simulink model "PILAN2021a"  (R2021a)
settings: Solver=FixedStepAuto  StartTime=0.0  StopTime=41.24  FixedStep=0.001  RelTol=1e-3  EnableMultiTasking=on
values from neighbouring files (symbols this model uses):
  den_lpf_d = den_lpf20    [Mainframe_init.m]    (also in load_autopilot.m)
  Emulated_FCC_IO_Delay = 7    [Mainframe_init.m]
  Enable_Gyros = 0    [Mainframe_init.m]
  Enable_INS = 0    [Mainframe_init.m]
  num_lpf_d = num_lpf20    [Mainframe_init.m]    (also in load_autopilot.m)
undefined symbols (not defined in the file or in its folder): act_dmp, act_omega, Actuator, Aerodynamics, aMode, Autopilot, AUX, c_b_WGS, c_be, c_flat, c_grav, c_h_geop0, c_h_geope, c_pa0, c_pe, c_r0, c_rot, c_rsma, c_Tmp0, d_siB_0, d_siB_max, d_siB_min, dd_siB_max, dd_siB_min, dev, DiscIntNeverNeededParam, e_pa, e_Tmp, Earth, fin_maxrate, flag_I_act_switch, flag_I_aero_switch, flag_I_flat, flag_I_gravity_switch, flag_I_rot, Flight_Logic, hcr, HIL_Data, JMMM_0, JMMM_e, JSPB_e, lat_0, lon_0, Mass_Props, mB_0, mM_0, mM_e, National_Instruments, pBII_0, PCIe, pMPB, pNPB, propellant_kg, prp_FBPB, prp_mdot, prp_T, pSPB, pwm_output1, qEG_0, qIB_0 ... (+30)
libraries: simulink x42, simulink_extras x24, aerolibcommonsys x4, px4lib x2, custom_blocks x1, dspstat3 x1, pil_lib x1, aerolibtransform2 x1, sldrtlib x1, aerolibnav x1
(part 1 of 16)
settings Model: CodeVerificationMode=processor-in-the-loop (pil)  ExtModeTrigDuration=10  Creator=m.hiepp  LastModifiedBy=sasson
settings SolverCC: AlgebraicLoopSolver=TrustRegion  PositivePriorityOrder=on  AutoInsertRateTranBlk=on
settings DataIOCC: SignalLogging=off  ReturnWorkspaceOutputs=off
settings OptimizationCC: EnhancedBackFolding=on  PassReuseOutputArgsAs=Individual arguments  ZeroExternalMemoryAtStartup=off  ZeroInternalMemoryAtStartup=off  MaxStackSize=64  OptimizeBlockOrder=speed  DifferentSizesBufferReuse=on  OptimizationCustomize=off  EfficientTunableParamExpr=on
settings DebuggingCC: ParameterPrecisionLossMsg=none  ParameterTunabilityLossMsg=error  SFMachineParentedDataDiag=warning  UnderSpecifiedDimensionMsg=warning  ArithmeticOperatorsInVariantConditions=warning
settings HardwareCC: ProdBitPerPointer=32  ProdBitPerSizeT=32  ProdBitPerPtrDiffT=32  ProdLargestAtomicInteger=Long  ProdLargestAtomicFloat=Double  ProdWordSize=32  ProdLongLongMode=on  ProdHWDeviceType=ARM Compatible->ARM Cortex
settings SFSimCC: MATLABDynamicMemAlloc=off  CustomCodeUndefinedFunction=UseInterfaceOnly  SimTargetLang=C++
settings RTWCC: SystemTargetFile=ert.tlc  HardwareBoard=PX4 Pixhawk 2.1 (Cube)  TLCOptions="-aInlineSetEventsForThisBaseRateFcn=TLC_FALSE -aSuppressMultiTaskScheduler=TLC_FALSE  -aRateBasedStepFcn=0"  TemplateMakefile=ert_default_tmf  GenerateReport=on  Toolchain=GNU Tools for PX4 Autopilots  IncludeHyperlinkInReport=on  LaunchReport=on  PortableWordSizes=on  CreateSILPILBlock=PIL  TargetLang=C++  GenerateTraceInfo=on  GenerateTraceReport=on  GenerateTraceReportSl=on  GenerateTraceReportSf=on  GenerateTraceReportEml=on
settings CodeAppCC: ForceParamTrailComments=on  IgnoreCustomStorageClasses=off  MaxIdLength=95  OperatorAnnotations=on  SimulinkDataObjDesc=on  SFDataObjDesc=on  InsertBlockDesc=on
settings ERTTargetCC: SupportContinuousTime=on  ExtModeTransport=3  ExtModeStaticAlloc=on  ExtModeStaticAllocSize=1024  ExtModeMexFile=ext_xcp  ExtModeIntrfLevel=Level2 - Open

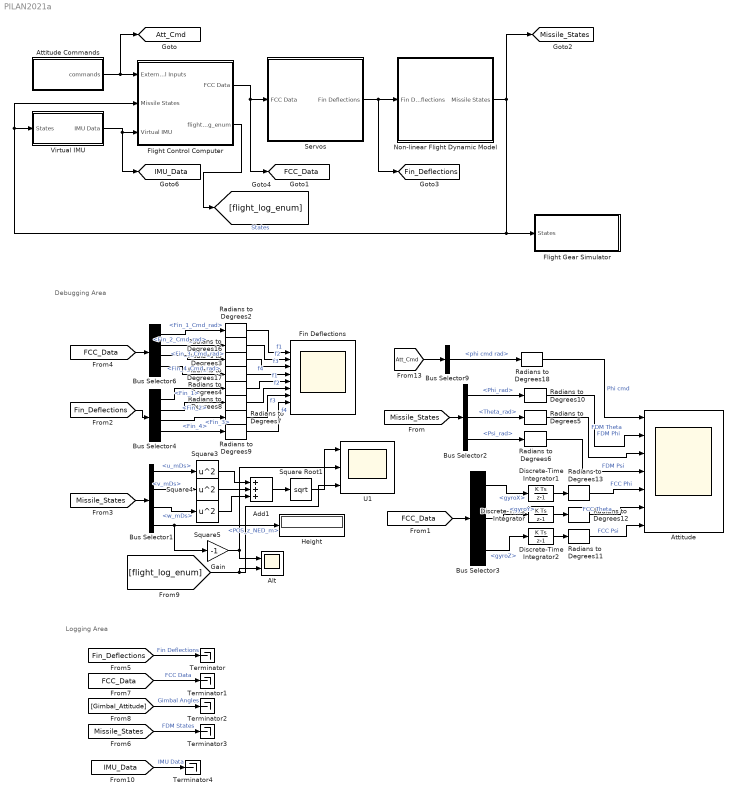
== system PILAN2021a ==
  note: Debugging Area
  note: Logging Area
  Add1 : Sum  Inputs=+++
  Alt : Scope  NumInputPorts=2
  Attitude : Scope  NumInputPorts=7
  Attitude Commands : Subsystem
  Bus Selector1 : BusSelector  OutputSignals=Translation_States.u_mDs,Translation_States.v_mDs,Translation_States.w_mDs,POS_NED.POS_z_NED_m
  Bus Selector2 : BusSelector  OutputSignals=Attitude_States.ATT_Euler.Phi_rad,Attitude_States.ATT_Euler.Theta_rad,Attitude_States.ATT_Euler.Psi_rad
  Bus Selector3 : BusSelector  OutputSignals=Internal Data.gyroX,Internal Data.gyroY,Internal Data.gyroZ
  Bus Selector4 : BusSelector  OutputSignals=Fin_1,Fin_2,Fin_3,Fin_4
  Bus Selector6 : BusSelector  OutputSignals=Control Surface Cmd.Fin_1_Cmd_rad,Control Surface Cmd.Fin_2_Cmd_rad,Control Surface Cmd.Fin_3_Cmd_rad,Control Surface Cmd.Fin_4_Cmd_rad
  Bus Selector9 : BusSelector  OutputSignals=phi cmd rad
  Discrete-Time Integrator : DiscreteIntegrator  SampleTime=0.01  ICPrevOutput=DiscIntNeverNeededParam  ICPrevScaledInput=DiscIntNeverNeededParam
  Discrete-Time Integrator1 : DiscreteIntegrator  SampleTime=0.01  ICPrevOutput=DiscIntNeverNeededParam  ICPrevScaledInput=DiscIntNeverNeededParam
  Discrete-Time Integrator2 : DiscreteIntegrator  SampleTime=0.01  ICPrevOutput=DiscIntNeverNeededParam  ICPrevScaledInput=DiscIntNeverNeededParam
  Fin Deflections : Scope  NumInputPorts=8
  Flight Control Computer : Subsystem  VariantControl=VSS_FCC_REAL
  Flight Gear Simulator : Subsystem  Variant=on
  Gain : Gain  Gain=-1
  Height : Display
  Non-linear Flight Dynamic Model : Subsystem  VariantControl=VSS_FDM_SOPH
      mask init:
      | load('generated_FDM_params')
  Radians to Degrees{2..13,16..18} (15 alike) : simulink_extras/Transformations/Radians to Degrees
  Servos : Subsystem  Variant=on
  Square Root1 : Sqrt  SaturateOnIntegerOverflow=on
  Square3 : Math  Operator=square  SaturateOnIntegerOverflow=on
  Square4 : Math  Operator=square  SaturateOnIntegerOverflow=on
  Square5 : Math  Operator=square  SaturateOnIntegerOverflow=on
  Terminator{,1..4} (5 alike) : Terminator
  U1 : Scope  NumInputPorts=3
  Virtual IMU : Subsystem
  tag scope: Att_Cmd=global, FCC_Data=global, Fin_Deflections=global, IMU_Data=global, Missile_States=global
  wires:
  [IMU_Data] -> Terminator4/1  "IMU Data"
  Bus Selector3/2 -> Discrete-Time Integrator/1  "<gyroY>"
  Discrete-Time Integrator1/1 -> Radians to Degrees13/1
  Radians to Degrees11/1 -> Attitude/7  "FCC Psi"
  Discrete-Time Integrator/1 -> Radians to Degrees12/1
  [FCC_Data] -> Bus Selector6/1
  Bus Selector1/4 -> Gain/1, Height/1  "<POS_z_NED_m>"
  Flight Control Computer/1(FCC Data) -> [FCC_Data], Servos/1(FCC Data)
  Radians to Degrees2/1 -> Fin Deflections/1  "f1"
  Radians to Degrees4/1 -> Fin Deflections/5  "f1"
  Radians to Degrees18/1 -> Attitude/1  "Phi cmd"
  Bus Selector6/1 -> Radians to Degrees2/1  "<Fin_1_Cmd_rad>"
  Radians to Degrees3/1 -> Fin Deflections/3  "f3"
  Radians to Degrees17/1 -> Fin Deflections/4  "f4"
  Radians to Degrees13/1 -> Attitude/5  "FCC Phi"
  [Missile_States] -> Bus Selector1/1
  Bus Selector3/1 -> Discrete-Time Integrator1/1  "<gyroX>"
  Discrete-Time Integrator2/1 -> Radians to Degrees11/1
  [Gimbal_Attitude] -> Terminator2/1  "Gimbal Angles"
  [FCC_Data] -> Terminator1/1  "FCC Data"
  Square5/1 -> Add1/3
  Bus Selector6/2 -> Radians to Degrees16/1  "<Fin_2_Cmd_rad>"
  [Fin_Deflections] -> Terminator/1  "Fin Deflections"
  Bus Selector6/4 -> Radians to Degrees17/1  "<Fin_4_Cmd_rad>"
  Square3/1 -> Add1/1
  Bus Selector1/1 -> Square3/1  "<u_mDs>"
  Add1/1 -> Square Root1/1
  Radians to Degrees6/1 -> Attitude/4  "FDM Psi"
  Bus Selector4/4 -> Radians to Degrees9/1  "<Fin_4>"
  Virtual IMU/1(" IMU Data") -> [IMU_Data], Flight Control Computer/3(Virtual IMU)
  Radians to Degrees10/1 -> Attitude/2  "FDM Phi"
  Bus Selector1/3 -> Square5/1  "<w_mDs>"
  Bus Selector1/2 -> Square4/1  "<v_mDs>"
  Radians to Degrees5/1 -> Attitude/3  "FDM Theta"
  Non-linear Flight Dynamic Model/1(Missile States) -> Flight Control Computer/2(Missile States), Virtual IMU/1(States), Flight Gear Simulator/1(States), [Missile_States]  "States"
  Bus Selector9/1 -> Radians to Degrees18/1  "<phi cmd rad>"
  Square4/1 -> Add1/2
  [Missile_States] -> Bus Selector2/1
  Bus Selector2/2 -> Radians to Degrees5/1  "<Theta_rad>"
  Bus Selector6/3 -> Radians to Degrees3/1  "<Fin_3_Cmd_rad>"
  Servos/1(Fin Deflections) -> [Fin_Deflections], Non-linear Flight Dynamic Model/1(Fin Deflections)
  Radians to Degrees16/1 -> Fin Deflections/2  "f2"
  Radians to Degrees9/1 -> Fin Deflections/8  "f4"
  Attitude Commands/1(commands) -> [Att_Cmd], Flight Control Computer/1(External Inputs)
  Radians to Degrees8/1 -> Fin Deflections/6  "f2"
  Bus Selector3/3 -> Discrete-Time Integrator2/1  "<gyroZ>"
  Bus Selector2/3 -> Radians to Degrees6/1  "<Psi_rad>"
  Bus Selector4/3 -> Radians to Degrees7/1  "<Fin_3>"
  Radians to Degrees7/1 -> Fin Deflections/7  "f3"
  Bus Selector2/1 -> Radians to Degrees10/1  "<Phi_rad>"
  [Att_Cmd] -> Bus Selector9/1
  [Missile_States] -> Terminator3/1  "FDM States"
  [Fin_Deflections] -> Bus Selector4/1
  Radians to Degrees12/1 -> Attitude/6  "FCC Theta"
  Bus Selector4/1 -> Radians to Degrees4/1  "<Fin_1>"
  [FCC_Data] -> Bus Selector3/1
  Square Root1/1 -> U1/1
  Bus Selector4/2 -> Radians to Degrees8/1  "<Fin_2>"
  Gain/1 -> Alt/1, U1/2
  Flight Control Computer/2(flight_log_enum) -> [flight_log_enum]
  [flight_log_enum] -> U1/3, Alt/2

== system PILAN2021a/Attitude Commands ==
  Bus Creator : BusCreator  Inputs=3
  Delayed Sine : custom_blocks/Delayed Sine  amp=deg2rad(65)  bias=0  freq=pi/3  phase=0  onTime=5  duration=3
  Enabled Subsystem1 : Subsystem  TreatAsAtomicUnit=on
  Radians to Degrees : simulink_extras/Transformations/Radians to Degrees
  Scope : Scope
  Zero : Constant  Value=0  OutDataTypeStr=Inherit: Inherit via back propagation
  Zero1 : Constant  Value=0  OutDataTypeStr=Inherit: Inherit via back propagation
  commands : Outport
  wires:
  Delayed Sine/1 -> Radians to Degrees/1, Bus Creator/1  "phi cmd rad"
  Bus Creator/1 -> commands/1
  Zero/1 -> Bus Creator/3  "psi cmd rad"
  Zero1/1 -> Bus Creator/2  "theta cmd rad"
  Enabled Subsystem1/1(CalibrationTime) -> Delayed Sine/1  "Calibration Time"
  [HIL_Ready] -> Enabled Subsystem1/Trigger
  Radians to Degrees/1 -> Scope/1

== system PILAN2021a/Flight Control Computer ==
  External Inputs : Inport
  Missile States : Inport  Port=2
  Virtual IMU : Inport  Port=3
  Bus Creator : BusCreator  Inputs=2
  Bus Selector : BusSelector  OutputSignals=signal1,flight_mode_enum
  Constant1 : Constant  Value=Enable_Gyros  OutDataTypeStr=single
  Constant4 : Constant  Value=Enable_INS  OutDataTypeStr=single
  Debug : Scope
  FCC - Real or Emulated : Subsystem  Variant=on
  FCC_SYNC : Scope
  Heartbeat Check : Subsystem
  Recieve from FCC : Subsystem
  Send to FCC : Subsystem
  FCC Data : Outport
  flight_log_enum : Outport  Port=2
  wires:
  Constant4/1 -> Send to FCC/1(Enable INS Flag)
  Recieve from FCC/2(internal data) -> Bus Creator/2  "Internal Data"
  Recieve from FCC/1(fin_cmd_rad) -> Bus Creator/1  "Control Surface Cmd"
  External Inputs/1 -> Send to FCC/5(External Inputs)
  Missile States/1 -> Send to FCC/3(Missile States)
  Send to FCC/1(data out) -> FCC - Real or Emulated/1(Input Data)
  Recieve from FCC/3(Other) -> Debug/1
  Constant1/1 -> Send to FCC/2(Enable Gyros Flag)
  Heartbeat Check/1(Communication Delay) -> FCC_SYNC/1
  Bus Creator/1 -> FCC Data/1  "FCC data"
  Virtual IMU/1 -> Send to FCC/4(Virtual IMU)
  Send to FCC/2(Heartbeat Send) -> [Heartbeat_Sent]
  Recieve from FCC/4(HeartBeat_recived) -> [Heartbeat_Received]
  [Heartbeat_Sent] -> Heartbeat Check/1(Send)
  [Heartbeat_Received] -> Heartbeat Check/2(receive)  "receive"
  FCC - Real or Emulated/1(Output Data) -> Bus Selector/1
  Bus Selector/1 -> Recieve from FCC/1(data in)  "<signal1>"
  Bus Selector/2 -> flight_log_enum/1  "<flight_mode_enum>"

== system PILAN2021a/Flight Gear Simulator ==
  States : Inport
  Flight Simulator Off : Subsystem  VariantControl=VSS_FLIGHTGEAR_OFF
  Flight Simulator On : Subsystem  VariantControl=VSS_FLIGHTGEAR_ON

== system PILAN2021a/Non-linear Flight Dynamic Model ==
  Fin Deflections : Inport
  Environment : Subsystem
  Extract States : Subsystem
  GRM_Airframe : Subsystem
      mask Display: image('$imagefile'); % Use "Edit Image" on toolstrip to change.
  Stop-Condition : Subsystem
  Subsystem1 : Subsystem  Commented=on
  Translate Fins : Subsystem
  Missile States : Outport  VectorParamsAs1DForOutWhenUnconnected=off
  wires:
  Fin Deflections/1 -> Translate Fins/1(Servo Deflections)
  Extract States/1(States) -> Missile States/1, Stop-Condition/1(States)  "States"
  Translate Fins/1(afinB) -> GRM_Airframe/1(siB_cmd)
  GRM_Airframe/1(airfr) -> Extract States/1(airfr_bus)
  Environment/1(env_glbl_bus) -> GRM_Airframe/2(T_sim_glbl)

== system PILAN2021a/Servos ==
  FCC Data : Inport
  Emulated Servos : Subsystem  VariantControl=VSS_SERVOS_OFF
  Real Servos : Subsystem  VariantControl=VSS_SERVOS_ON
  Fin Deflections : Outport

== system PILAN2021a/Virtual IMU ==
  States : Inport
  Bus Creator1 : BusCreator  Inputs=3
  Bus Creator10 : BusCreator  Inputs=2
  Bus Creator2 : BusCreator  Inputs=3
  Bus Selector : BusSelector  OutputSignals=Translation_States_Dot.u_dot_mDs2,Translation_States_Dot.v_dot_mDs2,Translation_States_Dot.w_dot_mDs2,Rotation_States.p_radDs,Rotation_States.q_radDs,Rotation_States.r_radDs,Rotation_States_Dot.p_dot_radDs2,Rotation_States_Dot.q_dot_radDs2,Rotation_States_Dot.r_dot_radDs2,Attitude_States.ATT_Euler.Phi_rad,Attitude_States.ATT_Euler.Theta_rad
  Constant1 : Constant  Value=[0,0,0]
  Demux8 : Demux  Outputs=3
  Demux9 : Demux  Outputs=3
  Gravity Vector : Subsystem
  Mux1 : Mux  Inputs=3
  Mux2 : Mux  Inputs=3
  Mux3 : Mux  Inputs=3
  Three-axis Inertial Measurement Unit : aerolibnav/Three-axis Inertial Measurement Unit  units=Metric (MKS)  imu=[0.43197 -0.00245 -0.01265]  i_Ts=0  dtype_a=on  w_a=190  z_a=0.707  a_sf_cc=[1.00135 0.0029375 0.00018125; -0.0029375 1.001525 0.0025625; -0.00018125 -0.0025625 1.004375]  a_bias=[0.086853 0.0258 -0.009194]  a_sat="[-156.921  -156.921  -156.921  156.921 156.921 156.921]"  dtype_g=on  w_g=190  z_g=0.707  g_sf_cc=[1.0045125 0.0045875 -0.005975; -0.0045875 1.0017125 0.0036875; 0.005975 -0.0036875 1.00243125]  g_bias=[-0.02167 0.011301 0.00202676]  g_sens=[0.000062068 0.0000443968 -0.0010608]  g_sat="[-34.9  -34.9  -34.9  34.9 34.9 34.9]"  i_rand=off  i_seeds=[23093 23094 23095 23096 23097 23098]  i_pow=[0.001 0.001 0.001 0.0001 0.0001 0.0001]
  " IMU Data" : Outport  VectorParamsAs1DForOutWhenUnconnected=off
  wires:
  Bus Selector/5 -> Mux2/2  "<q_radDs>"
  Mux3/1 -> Three-axis Inertial Measurement Unit/3
  Bus Selector/3 -> Mux1/3  "<w_dot_mDs2>"
  Bus Creator10/1 -> " IMU Data"/1  "Virtual IMU"
  Bus Selector/6 -> Mux2/3  "<r_radDs>"
  States/1 -> Bus Selector/1
  Bus Selector/11 -> Gravity Vector/2(Theta)  "<Theta_rad>"
  Bus Selector/2 -> Mux1/2  "<v_dot_mDs2>"
  Three-axis Inertial Measurement Unit/2 -> Demux9/1
  Bus Creator2/1 -> Bus Creator10/2  "gyro"
  Mux1/1 -> Three-axis Inertial Measurement Unit/1
  Mux2/1 -> Three-axis Inertial Measurement Unit/2
  Demux8/3 -> Bus Creator1/3  "accZ"
  Demux9/2 -> Bus Creator2/2  "gyroY"
  Demux9/1 -> Bus Creator2/1  "gyroX"
  Three-axis Inertial Measurement Unit/1 -> Demux8/1
  Demux8/1 -> Bus Creator1/1  "accX"
  Constant1/1 -> Three-axis Inertial Measurement Unit/4
  Bus Selector/4 -> Mux2/1  "<p_radDs>"
  Bus Creator1/1 -> Bus Creator10/1  "accelerometer"
  Demux8/2 -> Bus Creator1/2  "accY"
  Bus Selector/1 -> Mux1/1  "<u_dot_mDs2>"
  Gravity Vector/1(g) -> Three-axis Inertial Measurement Unit/5
  Demux9/3 -> Bus Creator2/3  "gyroZ"
  Bus Selector/10 -> Gravity Vector/1(Phi)  "<Phi_rad>"
  Bus Selector/8 -> Mux3/2  "<q_dot_radDs2>"
  Bus Selector/7 -> Mux3/1  "<p_dot_radDs2>"
  Bus Selector/9 -> Mux3/3  "<r_dot_radDs2>"

== system PILAN2021a/Attitude Commands/Enabled Subsystem1 ==
  Trigger : TriggerPort  VariantControl=Variant  PortDimensions=1
  Digital Clock : DigitalClock  SampleTime=-1
  CalibrationTime : Outport  InitialOutput=1e9
  wires:
  Digital Clock/1 -> CalibrationTime/1

== system PILAN2021a/Flight Control Computer/FCC - Real or Emulated ==
  Input Data : Inport
  Emulated FCC : Subsystem  VariantControl=VSS_FCC_EMUL
  Real FCC : Subsystem  VariantControl=VSS_FCC_REAL
  Output Data : Outport

== system PILAN2021a/Flight Control Computer/Heartbeat Check ==
  note: This block ensures the Pixhawk is connected and functioning correctly
  Send : Inport
  receive : Inport  Port=2
  In Sync : Subsystem
  Communication Delay : Outport
  wires:
  Send/1 -> In Sync/1(send)
  receive/1 -> In Sync/2(receive)
  In Sync/1(Heartbeat Sync) -> Communication Delay/1

== system PILAN2021a/Flight Control Computer/Recieve from FCC ==
  data in : Inport
  Bus Creator1 : BusCreator  Inputs=12
  Bus Creator4 : BusCreator  Inputs=4
  Cast To Double{,1..17} (18 alike) : DataTypeConversion  OutDataTypeStr=double
  Demux : Demux  Outputs=18
  fin_cmd_rad : Outport  PortDimensions=4
  internal data : Outport  Port=2
  Other : Outport  Port=3
  HeartBeat_recived : Outport  Port=4
  wires:
  data in/1 -> Demux/1
  Demux/1 -> Cast To Double/1
  Demux/7 -> Cast To Double6/1  "gyroY"
  Demux/11 -> Cast To Double10/1  "w"
  Demux/10 -> Cast To Double9/1  "v"
  Demux/9 -> Cast To Double8/1  "u"
  Demux/8 -> Cast To Double7/1  "gyroZ"
  Demux/4 -> Cast To Double3/1  "Fin_3_Cmd_rad"
  Demux/5 -> Cast To Double4/1  "Fin_4_Cmd_rad"
  Demux/3 -> Cast To Double2/1  "Fin_2_Cmd_rad"
  Demux/2 -> Cast To Double1/1  "Fin_1_Cmd_rad"
  Demux/6 -> Cast To Double5/1  "gyroX"
  Bus Creator4/1 -> fin_cmd_rad/1
  Bus Creator1/1 -> internal data/1
  Cast To Double1/1 -> Bus Creator4/1  "Fin_1_Cmd_rad"
  Cast To Double2/1 -> Bus Creator4/2  "Fin_2_Cmd_rad"
  Cast To Double3/1 -> Bus Creator4/3  "Fin_3_Cmd_rad"
  Cast To Double4/1 -> Bus Creator4/4  "Fin_4_Cmd_rad"
  Cast To Double8/1 -> Bus Creator1/4  "u"
  Cast To Double9/1 -> Bus Creator1/5  "v"
  Cast To Double10/1 -> Bus Creator1/6  "w"
  Demux/12 -> Cast To Double12/1  "x"
  Demux/14 -> Cast To Double14/1  "z"
  Demux/15 -> Cast To Double15/1  "p"
  Demux/16 -> Cast To Double16/1  "q"
  Demux/17 -> Cast To Double11/1  "r"
  Demux/13 -> Cast To Double13/1  "y"
  Cast To Double12/1 -> Bus Creator1/7  "x"
  Cast To Double13/1 -> Bus Creator1/8  "y"
  Cast To Double14/1 -> Bus Creator1/9  "z"
  Demux/18 -> Cast To Double17/1
  Cast To Double17/1 -> Other/1  "debug"
  Cast To Double7/1 -> Bus Creator1/3  "gyroZ"
  Cast To Double6/1 -> Bus Creator1/2  "gyroY"
  Cast To Double5/1 -> Bus Creator1/1  "gyroX"
  Cast To Double15/1 -> Bus Creator1/10  "p"
  Cast To Double16/1 -> Bus Creator1/11  "q"
  Cast To Double11/1 -> Bus Creator1/12  "r"
  Cast To Double/1 -> HeartBeat_recived/1

== system PILAN2021a/Flight Control Computer/Send to FCC ==
  Enable INS Flag : Inport
  Enable Gyros Flag : Inport  Port=2
  Missile States : Inport  Port=3
  Virtual IMU : Inport  Port=4
  External Inputs : Inport  Port=5
  Bus Selector : BusSelector  OutputSignals=Translation_States.u_mDs,Translation_States.v_mDs,Translation_States.w_mDs,POS_NED.POS_x_NED_m,POS_NED.POS_y_NED_m,POS_NED.POS_z_NED_m,Rotation_States.p_radDs,Rotation_States.q_radDs,Rotation_States.r_radDs
  Bus Selector1 : BusSelector  OutputSignals=phi cmd rad
  Bus Selector2 : BusSelector  OutputSignals=accelerometer.accX,accelerometer.accY,accelerometer.accZ,gyro.gyroX,gyro.gyroY,gyro.gyroZ
  Bus Selector3 : BusSelector  OutputSignals=Attitude_States.ATT_Euler.Phi_rad,Attitude_States.ATT_Euler.Theta_rad,Attitude_States.ATT_Euler.Psi_rad
  Cast To Single{1..23} (23 alike) : DataTypeConversion  OutDataTypeStr=single
  Heartbeat Counter : Subsystem
  Mux : Mux  Inputs=23
  Scope : Scope
  data out : Outport
  Heartbeat Send : Outport  Port=2
  wires:
  Heartbeat Counter/1(Out1) -> Cast To Single18/1  "send"
  Enable INS Flag/1 -> Cast To Single17/1
  [HIL_Ready] -> Cast To Single19/1  "send"
  Mux/1 -> data out/1, Scope/1  "send"
  Missile States/1 -> Bus Selector3/1, Bus Selector/1
  Bus Selector1/1 -> Cast To Single20/1  "<phi cmd rad>"
  External Inputs/1 -> Bus Selector1/1
  Bus Selector/9 -> Cast To Single7/1  "<r_radDs>"
  Bus Selector2/1 -> Cast To Single6/1  "<accX>"
  Bus Selector2/2 -> Cast To Single5/1  "<accY>"
  Bus Selector2/3 -> Cast To Single4/1  "<accZ>"
  Bus Selector2/4 -> Cast To Single3/1  "<gyroX>"
  Bus Selector2/6 -> Cast To Single1/1  "<gyroZ>"
  Enable Gyros Flag/1 -> Cast To Single16/1
  Cast To Single1/1 -> Mux/19
  Bus Selector2/5 -> Cast To Single2/1  "<gyroY>"
  Cast To Single2/1 -> Mux/18
  Cast To Single3/1 -> Mux/17
  Cast To Single4/1 -> Mux/16
  Cast To Single5/1 -> Mux/15
  Cast To Single6/1 -> Mux/14
  Cast To Single7/1 -> Mux/13
  Cast To Single15/1 -> Mux/5
  Bus Selector/1 -> Cast To Single15/1  "<u_mDs>"
  Bus Selector/8 -> Cast To Single8/1  "<q_radDs>"
  Cast To Single8/1 -> Mux/12
  Cast To Single9/1 -> Mux/11
  Cast To Single10/1 -> Mux/10
  Cast To Single11/1 -> Mux/9
  Cast To Single12/1 -> Mux/8
  Cast To Single13/1 -> Mux/7
  Cast To Single14/1 -> Mux/6
  Bus Selector/2 -> Cast To Single14/1  "<v_mDs>"
  Bus Selector/3 -> Cast To Single13/1  "<w_mDs>"
  Bus Selector/4 -> Cast To Single12/1  "<POS_x_NED_m>"
  Bus Selector/5 -> Cast To Single11/1  "<POS_y_NED_m>"
  Bus Selector/6 -> Cast To Single10/1  "<POS_z_NED_m>"
  Bus Selector/7 -> Cast To Single9/1  "<p_radDs>"
  Cast To Single16/1 -> Mux/4
  Cast To Single17/1 -> Mux/3
  Cast To Single19/1 -> Mux/1
  Cast To Single20/1 -> Mux/23
  Bus Selector3/1 -> Cast To Single21/1  "<Phi_rad>"
  Cast To Single21/1 -> Mux/20
  Bus Selector3/3 -> Cast To Single23/1  "<Psi_rad>"
  Bus Selector3/2 -> Cast To Single22/1  "<Theta_rad>"
  Cast To Single22/1 -> Mux/21
  Cast To Single23/1 -> Mux/22
  Virtual IMU/1 -> Bus Selector2/1
  Cast To Single18/1 -> Heartbeat Send/1, Mux/2

== system PILAN2021a/Flight Gear Simulator/Flight Simulator Off ==
  States : Inport
  Terminator : Terminator
  wires:
  States/1 -> Terminator/1

== system PILAN2021a/Flight Gear Simulator/Flight Simulator On ==
  States : Inport
  Bus Creator : BusCreator  Inputs=3
  Bus Selector1 : BusSelector  OutputSignals=POS_NED.POS_x_NED_m,POS_NED.POS_y_NED_m,POS_NED.POS_z_NED_m,Attitude_States.ATT_Euler.Phi_rad,Attitude_States.ATT_Euler.Theta_rad,Attitude_States.ATT_Euler.Psi_rad
  Demux : Demux  Outputs=2
  Flat Earth to LLA : aerolibtransform2/Flat Earth to LLA  units=Metric (MKS)  ptype=Earth (WGS84)  F=1/298.257223563  R=6378137  refPosPort=off  LL0=[32.086241 34.768375]  psi=0
  FlightGear Preconfigured 6DoF Animation : Subsystem  TreatAsAtomicUnit=on  SimViewingDevice=on  mask(FlightGearQuick6DoFAnimation){xFlightGearVersion=v2018.3, DestinationIpAddress=127.0.0.1, DestinationPort=5502, SampleTime=0.001, packetVersion=24}
      mask prompts: xFlightGearVersion "aeroblks:aeroblkfltsims:blockFlightGearQuick6DoFAnimationParamFlightGearversion"; DestinationIpAddress "aeroblks:aeroblkfltsims:blockFlightGearQuick6DoFAnimationParamDestinationIPaddress"; DestinationPort "aeroblks:aeroblkfltsims:blockFlightGearQuick6DoFAnimationParamDestinationport"; SampleTime "aeroblks:aeroblkfltsims:blockFlightGearQuick6DoFAnimationParamSampletime1forinherited"; packetVersion "aeroblks:aeroblkfltsims:blockFlightGearPackNetParamFlightGearPacketversion"
      mask help: aeroblks:aeroblkfltsims:blockFlightGearQuick6DoFAnimationDesc
      mask init:
      | aeroicon('aeroblkfgsend');
      settings: AttributesFormatString=Version Selected: %<xFlightGearVersion>
      mask Help: eval('asbhelp(''flightgear_preconfigured_6dof_animation'')');
      mask TypeOptions xFlightGearVersion: aeroblks:aeroblkfltsims:blockFlightGearVersionCombov20 | aeroblks:aeroblkfltsims:blockFlightGearVersionCombov24 | aeroblks:aeroblkfltsims:blockFlightGearVersionCombov26 | aeroblks:aeroblkfltsims:blockFlightGearVersionCombov28 | aeroblks:aeroblkfltsims:blockFlightGearVersionCombov210 | aeroblks:aeroblkfltsims:blockFlightGearVersionCombov212 | aeroblks:aeroblkfltsims:blockFlightGearVersionCombov30 | aeroblks:aeroblkfltsims:blockFlightGearVersionCombov32 | aeroblks:aeroblkfltsims:blockFlightGearVersionCombov34 | aeroblks:aeroblkfltsims:blockFlightGearVersionCombov20161 | aeroblks:aeroblkfltsims:blockFlightGearVersionCombov20163 | aeroblks:aeroblkfltsims:blockFlightGearVersionCombov20171 | aeroblks:aeroblkfltsims:blockFlightGearVersionCombov20173 | aeroblks:aeroblkfltsims:blockFlightGearVersionCombov20181 | aeroblks:aeroblkfltsims:blockFlightGearVersionCombov20182 | aeroblks:aeroblkfltsims:blockFlightGearVersionCombov20183
      mask TypeOptions packetVersion: aeroblks:aeroblkfltsims:blockFlightGearPacketVersionCombo24
      mask DialogControl xFlightGearVersion Prompt: FlightGear version:
      mask DialogControl DestinationIpAddress Prompt: Destination IP address:
      mask DialogControl DestinationPort Prompt: Destination port:
      mask DialogControl SampleTime Prompt: Sample time (-1 for inherited):
      mask DialogControl packetVersion Prompt: FlightGear packet version:
      mask Display: port_label('input',1,'l,\mu,h,\phi,\theta,\psi','texmode','on')
  FlightGear1 : Subsystem  mask(FlightGear){}
      mask DialogControl Control2 Prompt: Please ensure you have FlightGear installed before proceeding
      mask DialogControl Control4 Prompt: Once FlightGear has finished loading you may minimize the terminal window and run the simulation
      mask DialogControl Control6 Prompt: Please note this feature is only supported in "normal mode"
      mask DialogControl Control5 Prompt: Launch
      mask DialogControl Control5 Callback:
      | simPath = which(bdroot);
      | idx = strfind(simPath,'\');
      | dirPath = simPath(1:idx(end));
      | LaunchFGPath = append(dirPath,'req\runfg.bat&');
      | system(LaunchFGPath)
      mask Display: disp("Launch\n FlightGear Simulator")
  Mux2 : Mux  Inputs=6
  ref : Constant  Value=-10  OutDataTypeStr=Inherit: Inherit via back propagation
  wires:
  Flat Earth to LLA/1 -> Demux/1
  Demux/1 -> Mux2/2
  States/1 -> Bus Selector1/1
  Bus Selector1/2 -> Bus Creator/2  "<POS_y_NED_m>"
  Demux/2 -> Mux2/1
  Bus Selector1/3 -> Bus Creator/3  "<POS_z_NED_m>"
  Bus Selector1/4 -> Mux2/4  "<Phi_rad>"
  Bus Selector1/6 -> Mux2/6  "<Psi_rad>"
  Bus Selector1/5 -> Mux2/5  "<Theta_rad>"
  Flat Earth to LLA/2 -> Mux2/3
  Mux2/1 -> FlightGear Preconfigured 6DoF Animation/1(In1)
  ref/1 -> Flat Earth to LLA/2
  Bus Creator/1 -> Flat Earth to LLA/1
  Bus Selector1/1 -> Bus Creator/1  "<POS_x_NED_m>"

== system PILAN2021a/Non-linear Flight Dynamic Model/Environment ==
  Add : Sum  Inputs=-+
  Bus Creator1 : BusCreator  Inputs=5
  Clock : Clock
  Constant6 : Constant  Value=T_sim_lnch
  Enabled Subsystem1 : Subsystem  TreatAsAtomicUnit=on
  From10 : From  Commented=on  GotoTag=HIL_Ready  TagVisibility=global
  Memory : Memory
  NOT : Logic  Operator=NOT  IconShape=distinctive  AllPortsSameDT=off  OutDataTypeStr=boolean
  atm_dynamic : Subsystem
  deviation_Tmp : Constant  Value=e_Tmp
  deviation_pa_QFH : Constant  Value=e_pa
  env_glbl_bus : Outport
  wires:
  atm_dynamic/1(vWEG) -> Bus Creator1/3
  Bus Creator1/1 -> env_glbl_bus/1  "env_glbl_bus"
  Clock/1 -> Add/2
  Constant6/1 -> Bus Creator1/2  "T_sim_lnch"
  deviation_pa_QFH/1 -> Bus Creator1/5  "e_pa"
  deviation_Tmp/1 -> Bus Creator1/4  "e_Tmp"
  From10/1 -> ?
  Add/1 -> Bus Creator1/1  "T_sim_glbl"
  Enabled Subsystem1/1(CalibrationTime) -> Add/1, NOT/1
  Memory/1 -> Enabled Subsystem1/Enable
  NOT/1 -> Memory/1

== system PILAN2021a/Non-linear Flight Dynamic Model/Extract States ==
  airfr_bus : Inport
  Assemble_States_Bus1 : Subsystem
  Bus Selector1 : BusSelector  OutputSignals=flight_dyn_bus.vBIB,flight_dyn_bus.wBIB,flight_dyn_bus.aBIB,flight_dyn_bus.d_wBIB,flight_dyn_bus.qIB,flight_dyn_bus.pBII,flight_dyn_bus.vBII
  MATLAB Function1 : MATLAB Function  TreatAsAtomicUnit=on
  quaternion_to_euler_angles1 : Subsystem
      mask help: transforms quaternions to Euler angles (roll, pitch, yaw)
      mask Help:
      | Name:
      | 
      |     quaternion_to_euler_angles
      | 
      | Description:
      | 
      |     This block implements the transformation of a quaternion into the
      |     corresponding Euler angles (zyx-sequence, roll, pitch, yaw).
      | 
      | Inputs  [size] [data type] [unit]:
      | 
      |     quaternion  [4] [double] [-]
      | 
      | Outputs  [size] [data type] [unit]:
      | 
      |     roll angle phi  [1] [double] [rad]
      |     pitch angle theta  [1] [double] [rad]
      |     yaw angle psi  [1] [double] [rad]
      mask Display:
      | %disp (' q --> (Phi,Theta,Psi) [rad]')
      | disp('q \rightarrow eu(\Phi;\Theta;\Psi)','texmode','on')
  States : Outport
  wires:
  Bus Selector1/6 -> Assemble_States_Bus1/6(POS_NED)  "<pBII>"
  quaternion_to_euler_angles1/1(eulx) -> Assemble_States_Bus1/5(Attitude_States)  "from Quat"
  MATLAB Function1/1(q_conj) -> quaternion_to_euler_angles1/1(q)
  Bus Selector1/5 -> MATLAB Function1/1(q)  "<qIB>"
  airfr_bus/1 -> Bus Selector1/1
  Bus Selector1/1 -> Assemble_States_Bus1/1(Translation_States)  "<vBIB>"
  Bus Selector1/2 -> Assemble_States_Bus1/2(Rotation_States)  "<wBIB>"
  Bus Selector1/4 -> Assemble_States_Bus1/4(Rotation_States_Dot)  "<d_wBIB>"
  Bus Selector1/3 -> Assemble_States_Bus1/3(Translation_States_Dot)  "<aBIB>"
  Assemble_States_Bus1/1(States) -> States/1
  Bus Selector1/7 -> Assemble_States_Bus1/7(POS_NED_dot)  "<vBII>"

== system PILAN2021a/Non-linear Flight Dynamic Model/GRM_Airframe ==
  siB_cmd : Inport
  T_sim_glbl : Inport  Port=2
  Bus Creator : BusCreator  Inputs=9
  aerodynamics : Subsystem
  environment : Subsystem
  fin_actuators : Subsystem
  forces_moments : Subsystem
  gravity : Subsystem
  input : Subsystem
  motion_kinematics : Subsystem
  propulsion : Subsystem
  rb_eom : Subsystem
  stream_flow : Subsystem
  weight_and_balance : Subsystem
  airfr : Outport  VectorParamsAs1DForOutWhenUnconnected=off
  wires:
  forces_moments/1(for_mom_bus) -> rb_eom/2(for_mom)
  [env] -> Bus Creator/9
  [fin] -> Bus Creator/7
  [motion_kin] -> Bus Creator/6
  [env_glbl] -> aerodynamics/4(env_glbl)
  aerodynamics/1(aero) -> forces_moments/1(aero), [aero]
  [motion_kin] -> rb_eom/1(mot_kin)
  weight_and_balance/1(wab) -> rb_eom/3(wab), gravity/2(wab), [wab], propulsion/2(wab)
  [wab] -> aerodynamics/3(wab)
  [str_flow] -> Bus Creator/5
  [motion_kin] -> forces_moments/2(motion_kin)
  motion_kinematics/1(motion_kin) -> stream_flow/2(motion_kin), [motion_kin]
  [grav] -> Bus Creator/3
  Bus Creator/1 -> airfr/1  "airfr_bus"
  [aero] -> Bus Creator/4
  environment/1(env) -> [env], stream_flow/3(env), gravity/1(env)
  [prp] -> forces_moments/4(prp)
  [prp] -> Bus Creator/8
  stream_flow/1(str_flow) -> [str_flow], aerodynamics/1(str_flow)
  input/1(cmd_bus) -> fin_actuators/1(cmd)
  [wab] -> Bus Creator/2
  gravity/1(grav) -> [grav], forces_moments/3(grav)
  T_sim_glbl/1 -> [env_glbl], environment/2(env_glbl), weight_and_balance/1(env_glb), propulsion/1(env_glbl)
  siB_cmd/1 -> input/1(siB_cmd)
  rb_eom/1(flight_dyn) -> environment/1(flight_dyn), motion_kinematics/1(flight_dyn), stream_flow/1(flight_dyn), Bus Creator/1
  fin_actuators/1(fin) -> [fin], aerodynamics/2(fin)
  propulsion/1(prp) -> [prp]

== system PILAN2021a/Non-linear Flight Dynamic Model/Stop-Condition ==
  States : Inport
  AND : Logic  Inputs=3  IconShape=distinctive  AllPortsSameDT=off  OutDataTypeStr=boolean
  Bus Selector1 : BusSelector  OutputSignals=POS_NED.POS_z_NED_m,POS_NED_dot.POS_z_NED_dot_m
  Compare To Constant : Subsystem  mask(Compare To Constant){relop=>, const=-700, OutDataTypeStr=boolean, ZeroCross=on}
      mask prompts: relop "Simulink:masks:Operator_MP"; const "Simulink:masks:ConstantValue_MP"; OutDataTypeStr "Simulink:masks:OutputDataType_MP"; ZeroCross "Simulink:masks:EnableZerocrossingDetection_MP"
      mask help: Simulink:masks:CompareToConstant_MD
      mask init:
      | blkName = gcb;
      | 
      | if strcmp(get_param(gcbh,'OutDataTypeStr'),'boolean')
      | 	setValue = 'boolean';
      | else
      | 	setValue = 'fixdt(0, 8)';
      | end
      | 
      | set_param([blkName,'/Compare'],'relop',relop, ...
      | 	'OutDataTypeStr', setValue, 'ZeroCross', ZeroCross);
      | 
      | str = [relop,' C']; %default
      | 
      | const_str = get_param(blkName, 'const');
      | const_val = str2num(const_str);
      | 
      | if isempty(const_val) %#ok<ST2NM>
      |     %Expression/Variable
      |     str = [relop, ' ', strtrim(const_str)];
      | else
      |     if length(const_val) == 1 
      |         if Simulink.data.isSupportedEnumClass(class(const_val))
      |             % Special Handling for Enumerations
      |             if Simulink.data.getEnumTypeInfo(class(const_val), 'AddClassNameToEnumNames')
      |                 str = [relop, ' ', strtrim(const_str)];
      |             else
      |                 str = [relop, ' ', char(const_val)];
      |             end
      |         elseif(isfloat(const_val) || isinteger(const_val) || islogical(const_val)) 
      |                 str = [relop, ' ', num2str(const_val)];
      |         end
      |     end
      | end
      mask TypeOptions relop: == | ~= | < | <= | >= | >
      mask TypeOptions OutDataTypeStr: Simulink:masks:uint8 | Simulink:masks:boolean
      mask Callback ZeroCross: sl('zeroCrossEnable', gcbh);
      mask Display: disp(str)
  Compare To Constant1 : Subsystem  mask(Compare To Constant){relop=>, const=0, OutDataTypeStr=boolean, ZeroCross=on}
      mask prompts: relop "Simulink:masks:Operator_MP"; const "Simulink:masks:ConstantValue_MP"; OutDataTypeStr "Simulink:masks:OutputDataType_MP"; ZeroCross "Simulink:masks:EnableZerocrossingDetection_MP"
      mask help: Simulink:masks:CompareToConstant_MD
      mask init: same as PILAN2021a/Non-linear Flight Dynamic Model/Stop-Condition/Compare To Constant
      mask TypeOptions relop: == | ~= | < | <= | >= | >
      mask TypeOptions OutDataTypeStr: Simulink:masks:uint8 | Simulink:masks:boolean
      mask Callback ZeroCross: sl('zeroCrossEnable', gcbh);
      mask Display: disp(str)
  From4 : From  Commented=on  GotoTag=HIL_Ready  TagVisibility=global
  Stop Simulation : Stop
  wires:
  Bus Selector1/1 -> Compare To Constant/1(u)  "<POS_z_NED_m>"
  States/1 -> Bus Selector1/1
  Compare To Constant/1(y) -> AND/2
  AND/1 -> Stop Simulation/1
  From4/1 -> AND/1
  Bus Selector1/2 -> Compare To Constant1/1(u)  "<POS_z_NED_dot_m>"
  Compare To Constant1/1(y) -> AND/3

== system PILAN2021a/Non-linear Flight Dynamic Model/Subsystem1 ==
  Control Surface Deflections : Inport
  Envoronment : Inport  Port=2
  Enable : EnablePort
  Extract States : Subsystem
  Fin Deflections : Subsystem
  GRM_Airframe : Subsystem
      mask Display: image('$imagefile'); % Use "Edit Image" on toolstrip to change.
  Missile States : Outport
  wires:
  GRM_Airframe/1(airfr) -> Extract States/1(airfr_bus)
  Control Surface Deflections/1 -> Fin Deflections/1(Servo Deflections)
  Envoronment/1 -> GRM_Airframe/2(T_sim_glbl)
  Extract States/1(States) -> Missile States/1
  Fin Deflections/1(afinB) -> GRM_Airframe/1(siB_cmd)

== system PILAN2021a/Non-linear Flight Dynamic Model/Translate Fins ==
  Servo Deflections : Inport
  Add : Sum
  Bus Selector : BusSelector  OutputSignals=Fin_1,Fin_2,Fin_3,Fin_4
  Constant1 : Constant  Value=unc_fin_def_roll
  Constant2 : Constant  Value=unc_fin_def_pitch
  Constant3 : Constant  Value=unc_fin_def_yaw
  Degrees to Radians : Subsystem  mask(DegreesToRadians){}
      mask help: SimulinkBlocks:simulink_extras:DegreesToRadians_MD
      mask Help: web([docroot '/simulink/ref_extras/degreestoradians.html'])
      mask Display: disp('D2R')
  Degrees to Radians1 : Subsystem  mask(DegreesToRadians){}
      mask help: SimulinkBlocks:simulink_extras:DegreesToRadians_MD
      mask Help: web([docroot '/simulink/ref_extras/degreestoradians.html'])
      mask Display: disp('D2R')
  Degrees to Radians2 : Subsystem  mask(DegreesToRadians){}
      mask help: SimulinkBlocks:simulink_extras:DegreesToRadians_MD
      mask Help: web([docroot '/simulink/ref_extras/degreestoradians.html'])
      mask Display: disp('D2R')
  Vector Concatenate : Concatenate  NumInputs=4
  Vector Concatenate1 : Concatenate  NumInputs=3
  control_allocation : Subsystem
  afinB : Outport
  wires:
  Degrees to Radians2/1(Radians out) -> Vector Concatenate1/3
  Vector Concatenate1/1 -> control_allocation/1(fin_cmd)  "fin_cmd"
  Constant1/1 -> Degrees to Radians/1(Degrees in)  "xi_cmd"
  Degrees to Radians1/1(Radians out) -> Vector Concatenate1/2
  Degrees to Radians/1(Radians out) -> Vector Concatenate1/1
  Constant3/1 -> Degrees to Radians2/1(Degrees in)  "ze_cmd"
  Constant2/1 -> Degrees to Radians1/1(Degrees in)  "et_cmd"
  Bus Selector/2 -> Vector Concatenate/2  "<Fin_2>"
  Servo Deflections/1 -> Bus Selector/1
  Bus Selector/1 -> Vector Concatenate/1  "<Fin_1>"
  Bus Selector/4 -> Vector Concatenate/4  "<Fin_4>"
  Vector Concatenate/1 -> Add/1
  Bus Selector/3 -> Vector Concatenate/3  "<Fin_3>"
  control_allocation/1(siB_cmd) -> Add/2
  Add/1 -> afinB/1  "siB_cmd"

== system PILAN2021a/Servos/Emulated Servos ==
  FCC Data : Inport
  Bus Creator : BusCreator  Inputs=4
  Bus Selector : BusSelector  OutputSignals=Control Surface Cmd.Fin_1_Cmd_rad,Control Surface Cmd.Fin_2_Cmd_rad,Control Surface Cmd.Fin_3_Cmd_rad,Control Surface Cmd.Fin_4_Cmd_rad
  Transfer Fcn{1..4} (4 alike) : TransferFcn  Numerator=33770  Denominator=[1 395.7 33770]
  Fin Deflections : Outport
  wires:
  FCC Data/1 -> Bus Selector/1
  Bus Selector/1 -> Transfer Fcn1/1  "<Fin_1_Cmd_rad>"
  Bus Selector/2 -> Transfer Fcn2/1  "<Fin_2_Cmd_rad>"
  Bus Selector/3 -> Transfer Fcn3/1  "<Fin_3_Cmd_rad>"
  Bus Selector/4 -> Transfer Fcn4/1  "<Fin_4_Cmd_rad>"
  Bus Creator/1 -> Fin Deflections/1
  Transfer Fcn1/1 -> Bus Creator/1  "Fin_1"
  Transfer Fcn2/1 -> Bus Creator/2  "Fin_2"
  Transfer Fcn3/1 -> Bus Creator/3  "Fin_3"
  Transfer Fcn4/1 -> Bus Creator/4  "Fin_4"

== system PILAN2021a/Servos/Real Servos ==
  FCC Data : Inport
  Bus Creator : BusCreator  Inputs=4
  Demux : Demux
  Encoder Input : sldrtlib/Encoder Input  SampleTime=0.001  MaxMissedTicks=10  ShowMissedTicks=off  YieldWhenWaiting=off  DrvName=National_Instruments/PCIe-6321  DrvAddress=4294967295  DrvOptions=[0 0 0 2 2 2 2]  Channels=1:4  QuadMode=3  IndexPulse=1  InputFilter=Inf  DataType=1
      settings: AttributesFormatString=National Instruments\nPCIe-6321 [auto]
  Reset Encoders : Subsystem
  Terminator : Terminator
  Ticks to rads : Gain  Gain=2*pi/4096
  Fin Deflections : Outport
  wires:
  Encoder Input/1 -> Ticks to rads/1
  FCC Data/1 -> Terminator/1
  Bus Creator/1 -> Fin Deflections/1
  Demux/3 -> Bus Creator/3  "Fin_3"
  Demux/2 -> Bus Creator/2  "Fin_2"
  Demux/1 -> Bus Creator/1  "Fin_1"
  Demux/4 -> Bus Creator/4  "Fin_4"
  [HIL_Ready] -> Reset Encoders/1(Reset Encoders)
  Ticks to rads/1 -> Reset Encoders/2(Encoder Readings)
  Reset Encoders/1(Fin Angles) -> Demux/1

== system PILAN2021a/Virtual IMU/Gravity Vector ==
  Phi : Inport
  Theta : Inport  Port=2
  Cos : Trigonometry
  Cos1 : Trigonometry
  Cos2 : Trigonometry  Operator=cos
  Cos3 : Trigonometry  Operator=cos
  Multiply : Gain  Gain=9.81
  Multiply1 : Gain  Gain=9.81
  Multiply2 : Gain  Gain=-9.81
  Product : Product
  Product1 : Product
  Vector Concatenate1 : Concatenate  NumInputs=3
  g : Outport
  wires:
  Vector Concatenate1/1 -> g/1
  Cos/1 -> Multiply2/1
  Product/1 -> Multiply/1
  Cos1/1 -> Product/1
  Theta/1 -> Cos/1, Cos2/1
  Multiply/1 -> Vector Concatenate1/2
  Phi/1 -> Cos3/1, Cos1/1
  Product1/1 -> Multiply1/1
  Multiply1/1 -> Vector Concatenate1/3
  Multiply2/1 -> Vector Concatenate1/1
  Cos2/1 -> Product1/1, Product/2
  Cos3/1 -> Product1/2

== system PILAN2021a/Flight Control Computer/FCC - Real or Emulated/Emulated FCC ==
  Input Data : Inport
  Bus Creator : BusCreator  Inputs=2
  Delay : Delay  DelayLength=Emulated_FCC_IO_Delay  SampleTime=0.001
  Delay1 : Delay  DelayLength=Emulated_FCC_IO_Delay  SampleTime=0.001
  pCKAN : Subsystem
  Output Data : Outport
  wires:
  Input Data/1 -> Delay/1
  Delay/1 -> pCKAN/1(Serial In)
  pCKAN/1(Serial Out) -> Delay1/1
  Bus Creator/1 -> Output Data/1  "FCC data"
  Delay1/1 -> Bus Creator/1
  pCKAN/2(flight_mode_enum) -> Bus Creator/2

== system PILAN2021a/Flight Control Computer/FCC - Real or Emulated/Real FCC ==
  Input Data : Inport
  Bus Creator : BusCreator  Inputs=2
  PixBlock2 : Subsystem  Commented=on
  pCKAN : Subsystem  DialogController=pil_create_dialog  LoadFcn=|
      | try
      |    if ~strcmp(rtw.pil.getPILVersion, '9.10 (R2021a)_15')
      |       set_param(gcb, 'DialogController', '');
      |       set_param(gcb, 'DialogControllerArgs', '');
      |    end
      | catch e
      |       set_param(gcb, 'DialogController', '');
      |       set_param(gcb, 'DialogControllerArgs', '');
      | end
      mask help: PIL:pil:XILBlockMaskDesc
      mask Display: disp('PIL');
  Output Data : Outport
  wires:
  Input Data/1 -> pCKAN/1(Serial In)
  pCKAN/1(Serial Out) -> Bus Creator/1
  pCKAN/2(flight_mode_enum) -> Bus Creator/2
  Bus Creator/1 -> Output Data/1  "FCC data"

== system PILAN2021a/Flight Control Computer/Heartbeat Check/In Sync ==
  note: This block ensures the Pixhawk is connected and functioning correctly
  send : Inport
  receive : Inport  Port=2
  Cast To Single : DataTypeConversion  OutDataTypeStr=single
  Mux : Mux  Inputs=2
  Rate Transition : RateTransition  OutPortSampleTime=0.001
  Rate Transition1 : RateTransition  OutPortSampleTime=0.001
  Heartbeat Sync : Outport
  wires:
  receive/1 -> Rate Transition1/1  "receive"
  send/1 -> Rate Transition/1
  Rate Transition/1 -> Mux/1
  Rate Transition1/1 -> Cast To Single/1
  Mux/1 -> Heartbeat Sync/1
  Cast To Single/1 -> Mux/2

== system PILAN2021a/Flight Control Computer/Send to FCC/Heartbeat Counter ==
  note: Starting the heartbeat at negative values prevents unwanted FCC behaviour on startup
  Cast To Double14 : DataTypeConversion  OutDataTypeStr=single
  Heartbeat : simulink/Sources/Counter Free-Running  NumBits=16  tsamp=-1
  Subtract : Sum  Inputs=+-
  Zero : Constant  Value=1000  OutDataTypeStr=Inherit: Inherit via back propagation
  Out1 : Outport
  wires:
  Heartbeat/1 -> Cast To Double14/1
  Zero/1 -> Subtract/2
  Cast To Double14/1 -> Subtract/1  "send"
  Subtract/1 -> Out1/1

== system PILAN2021a/Flight Gear Simulator/Flight Simulator On/FlightGear Preconfigured 6DoF Animation ==
  In1 : Inport
  Angle Conversion : Subsystem
  Angle Conversion1 : Subsystem
  Demux : Demux  Outputs=6
  Pack net_fdm Packet for FlightGear : S-Function  FunctionName=saerofgpacknetfdm  Parameters=packetVersion, 'on','off','off','off','off','off', SampleTime  SFunctionDeploymentMode=off  EnableBusSupport=off
  PacketSize : Constant  Value=408
  Rate Transition : RateTransition  Integrity=off  Deterministic=off  OutPortSampleTime=SampleTime
  Simulation Pace : S-Function  FunctionName=saeroclockpacer  Parameters=SimulationPace,SleepMode,OutputPaceError,SampleTime  SFunctionDeploymentMode=off  EnableBusSupport=off  mask(Simulation Pace){SimulationPace=1, SleepMode=MATLAB Thread, OutputPaceError=off, SampleTime=SampleTime}
      mask prompts: SimulationPace "aeroblks:aeroblkanimutils:blockSimulationPaceParamSimulationpacesimsecperclocksec"; SleepMode "aeroblks:aeroblkanimutils:blockSimulationPaceParamSleepmode"; OutputPaceError "aeroblks:aeroblkanimutils:blockSimulationPaceParamOutputpaceerrorsec"; SampleTime "aeroblks:aeroblkanimutils:blockSimulationPaceParamSampletime1forinherited"
      mask help: aeroblks:aeroblkanimutils:blockSimulationPaceDesc
      mask init:
      | aeroicon('aeroblkpacer');
      settings: AttributesFormatString=%<SimulationPace> sec/sec
      mask Help: eval('asbhelp');
      mask TypeOptions SleepMode: aeroblks:aeroblkanimutils:blockSimulationPaceParamComboOff | aeroblks:aeroblkanimutils:blockSimulationPaceParamComboMATLABThread | aeroblks:aeroblkanimutils:blockSimulationPaceParamComboBusyWait | aeroblks:aeroblkanimutils:blockSimulationPaceParamComboAuto
      mask DialogControl SimulationPace Prompt: Simulation pace (sim sec per clock sec):
      mask DialogControl SleepMode Prompt: Sleep mode:
      mask DialogControl OutputPaceError Prompt: Output pace error (sec)
      mask DialogControl SampleTime Prompt: Sample time (-1 for inherited):
      mask Display:
      | text(0.5,0.60,'Set','horizontalAlignment','center');
      | text(0.5,0.40,'Pace','horizontalAlignment','center');
  UDP Send : S-Function  FunctionName=saerofgsend  Parameters=DestinationIpAddress,DestinationPort,-1,SampleTime,0  SFunctionDeploymentMode=off  EnableBusSupport=off
  Unit Sys : UnitConfiguration  UnitSystemsStr=SI,SI (extended)  AllowAllUnitSystems=off
  toSingle1 : DataTypeConversion  OutDataTypeStr=single
  toSingle2 : DataTypeConversion  OutDataTypeStr=single
  toSingle3 : DataTypeConversion  OutDataTypeStr=single
  wires:
  Angle Conversion1/1(out) -> Pack net_fdm Packet for FlightGear/2
  Angle Conversion/1(out) -> Pack net_fdm Packet for FlightGear/1
  Rate Transition/1 -> Demux/1
  toSingle3/1 -> Pack net_fdm Packet for FlightGear/6
  toSingle2/1 -> Pack net_fdm Packet for FlightGear/5
  toSingle1/1 -> Pack net_fdm Packet for FlightGear/4
  Pack net_fdm Packet for FlightGear/1 -> UDP Send/1
  In1/1 -> Rate Transition/1
  Demux/1 -> Angle Conversion/1(in)
  Demux/2 -> Angle Conversion1/1(in)
  Demux/3 -> Pack net_fdm Packet for FlightGear/3
  Demux/4 -> toSingle1/1
  Demux/5 -> toSingle2/1
  Demux/6 -> toSingle3/1
  PacketSize/1 -> UDP Send/2

== system PILAN2021a/Flight Gear Simulator/Flight Simulator On/FlightGear1 ==

== system PILAN2021a/Non-linear Flight Dynamic Model/Environment/Enabled Subsystem1 ==
  Enable : EnablePort
  Digital Clock : DigitalClock  SampleTime=-1
  CalibrationTime : Outport  InitialOutput=0
  wires:
  Digital Clock/1 -> CalibrationTime/1

== system PILAN2021a/Non-linear Flight Dynamic Model/Environment/atm_dynamic ==
  Add : Sum
  Add1 : Sum
  Bus Creator : BusCreator  Inputs=1
  Constant1 : Constant  Value=0
  Vector Concatenate : Concatenate  NumInputs=3
  course_angle_uncertainty : Constant  Value=0
  course_angle_wind : Constant  Value=0
  trafo_around_z_axis : Subsystem  mask(Transformation um z-Achse){}
      mask help: Dieser Block transformiert einen Vektor vec1 durch eine Drehung des Referenzkoordinatensystems um die z-Achse und um den Winkel gamma (in rad) in den Vektor vec2
      mask Help:
      | Name:
      | 
      |    trafo_around_z_axis
      | 
      | Beschreibung:
      | 
      |    Dieser Block transformiert einen Vektor vec1 durch eine Drehung des
      |    Referenzkoordinatensystems um die z-Achse und um den Winkel gamma
      |    (in rad) in den Vektor vec2
      | 
      | Inputs   [dimension]  [data type] [unit]:
      | 
      |     vec1    [3] [double] [-]
      |     gamma   [1] [double] [rad]
      | 
      | Outputs  [dimension]  [data type] [unit]:
      | 
      |     vec2  [3] [double] [-]
  vWW : Constant  Value=0
  vWW_uncertainty : Constant  Value=0
  vWEG : Outport  VectorParamsAs1DForOutWhenUnconnected=off
  wires:
  Bus Creator/1 -> vWEG/1  "atm_dyn_bus"
  trafo_around_z_axis/1(vec2) -> Bus Creator/1  "vWEG"
  Add1/1 -> Vector Concatenate/1
  course_angle_uncertainty/1 -> Add/2
  Constant1/1 -> Vector Concatenate/2, Vector Concatenate/3
  vWW/1 -> Add1/2
  Vector Concatenate/1 -> trafo_around_z_axis/1(vec1)
  Add/1 -> trafo_around_z_axis/2(gamma)
  vWW_uncertainty/1 -> Add1/1
  course_angle_wind/1 -> Add/1
